simulink model "IEEE14_case"  (R2024b)
settings: Solver=FixedStepAuto  StartTime=0  StopTime=2  FixedStep=1e-7  RelTol=1e-3
values from neighbouring files (symbols this model uses):
  GFL_15_Bva = 0.009    [IEEE14_parameters.m]
  GFL_15_C_bus_pu = 7.179419    [IEEE14_parameters.m]
  GFL_15_f0 = 60    [IEEE14_parameters.m]
  GFL_15_I_id = 691.26967    [IEEE14_parameters.m]
  GFL_15_I_iq = 691.26967    [IEEE14_parameters.m]
  GFL_15_I_od = 45.2207    [IEEE14_parameters.m]
  GFL_15_I_oq = 45.2207    [IEEE14_parameters.m]
  GFL_15_I_pll = 0.78    [IEEE14_parameters.m]
  GFL_15_Kdi = 0.09    [IEEE14_parameters.m]
  GFL_15_Kdo = 0.9    [IEEE14_parameters.m]
  GFL_15_Kqi = 0.09    [IEEE14_parameters.m]
  GFL_15_Kqo = 0.9    [IEEE14_parameters.m]
  GFL_15_Lg_pu = 0.631447    [IEEE14_parameters.m]
  GFL_15_mode = 1    [IEEE14_parameters.m]
  GFL_15_P_id = 3.7166    [IEEE14_parameters.m]
  GFL_15_P_iq = 3.7166    [IEEE14_parameters.m]
  GFL_15_P_od = 0.4798    [IEEE14_parameters.m]
  GFL_15_P_oq = 0.4798    [IEEE14_parameters.m]
  GFL_15_P_pll = 290.42    [IEEE14_parameters.m]
  GFL_15_Qe_ref = 0.2    [IEEE14_parameters.m]
  GFL_15_Rg_pu = 0.024016    [IEEE14_parameters.m]
  GFL_15_Sbase = 1.000000e+4    (= 10000)    [IEEE14_parameters.m]
  GFL_15_Tdi = 0.01    [IEEE14_parameters.m]
  GFL_15_Tdo = 0.2    [IEEE14_parameters.m]
  GFL_15_Tqi = 0.01    [IEEE14_parameters.m]
  GFL_15_Tqo = 0.2    [IEEE14_parameters.m]
  GFL_15_Vbase = 380    [IEEE14_parameters.m]
  GFL_15_Vdc_ref = 1.011475    [IEEE14_parameters.m]
  GFL_15_Vdcbase = 700    [IEEE14_parameters.m]
  GFL_15_vq_ref = 0    [IEEE14_parameters.m]
  GFL_16_Bva = 0.002    [IEEE14_parameters.m]
  GFL_16_C_bus_pu = 7.179419    [IEEE14_parameters.m]
  GFL_16_f0 = 60    [IEEE14_parameters.m]
  GFL_16_I_id = 691.26967    [IEEE14_parameters.m]
  GFL_16_I_iq = 691.26967    [IEEE14_parameters.m]
  GFL_16_I_od = 45.2207    [IEEE14_parameters.m]
  GFL_16_I_oq = 45.2207    [IEEE14_parameters.m]
  GFL_16_I_pll = 0.78    [IEEE14_parameters.m]
  GFL_16_Kdi = 0.05    [IEEE14_parameters.m]
  GFL_16_Kdo = 0.5    [IEEE14_parameters.m]
  GFL_16_Kqi = 0.05    [IEEE14_parameters.m]
  GFL_16_Kqo = 0.5    [IEEE14_parameters.m]
  GFL_16_Lg_pu = 0.631447    [IEEE14_parameters.m]
  GFL_16_mode = 1    [IEEE14_parameters.m]
  GFL_16_P_id = 3.7166    [IEEE14_parameters.m]
  GFL_16_P_iq = 3.7166    [IEEE14_parameters.m]
  GFL_16_P_od = 0.4798    [IEEE14_parameters.m]
  GFL_16_P_oq = 0.4798    [IEEE14_parameters.m]
  GFL_16_P_pll = 290.42    [IEEE14_parameters.m]
  GFL_16_Qe_ref = 0.2    [IEEE14_parameters.m]
  GFL_16_Rg_pu = 0.024016    [IEEE14_parameters.m]
  GFL_16_Sbase = 1.000000e+4    (= 10000)    [IEEE14_parameters.m]
  GFL_16_Tdi = 0.01    [IEEE14_parameters.m]
  GFL_16_Tdo = 0.2    [IEEE14_parameters.m]
  GFL_16_Tqi = 0.01    [IEEE14_parameters.m]
  GFL_16_Tqo = 0.2    [IEEE14_parameters.m]
  GFL_16_Vbase = 380    [IEEE14_parameters.m]
  GFL_16_Vdc_ref = 1.01144    [IEEE14_parameters.m]
  GFL_16_Vdcbase = 700    [IEEE14_parameters.m]
  GFL_16_vq_ref = 0    [IEEE14_parameters.m]
  GFL_17_Bva = 0.002    [IEEE14_parameters.m]
  GFL_17_C_bus_pu = 7.179419    [IEEE14_parameters.m]
  GFL_17_f0 = 60    [IEEE14_parameters.m]
  GFL_17_I_id = 691.26967    [IEEE14_parameters.m]
  GFL_17_I_iq = 691.26967    [IEEE14_parameters.m]
  GFL_17_I_od = 45.2207    [IEEE14_parameters.m]
  GFL_17_I_oq = 45.2207    [IEEE14_parameters.m]
  GFL_17_I_pll = 0.78    [IEEE14_parameters.m]
  GFL_17_Kdi = 0.05    [IEEE14_parameters.m]
  GFL_17_Kdo = 0.5    [IEEE14_parameters.m]
  GFL_17_Kqi = 0.05    [IEEE14_parameters.m]
  GFL_17_Kqo = 0.5    [IEEE14_parameters.m]
  GFL_17_Lg_pu = 0.631447    [IEEE14_parameters.m]
  GFL_17_mode = 1    [IEEE14_parameters.m]
  GFL_17_P_id = 3.7166    [IEEE14_parameters.m]
  GFL_17_P_iq = 3.7166    [IEEE14_parameters.m]
  GFL_17_P_od = 0.4798    [IEEE14_parameters.m]
  GFL_17_P_oq = 0.4798    [IEEE14_parameters.m]
  GFL_17_P_pll = 290.42    [IEEE14_parameters.m]
  GFL_17_Qe_ref = 0.2    [IEEE14_parameters.m]
  GFL_17_Rg_pu = 0.024016    [IEEE14_parameters.m]
  GFL_17_Sbase = 1.000000e+4    (= 10000)    [IEEE14_parameters.m]
  GFL_17_Tdi = 0.01    [IEEE14_parameters.m]
  GFL_17_Tdo = 0.2    [IEEE14_parameters.m]
  GFL_17_Tqi = 0.01    [IEEE14_parameters.m]
  GFL_17_Tqo = 0.2    [IEEE14_parameters.m]
  GFL_17_Vbase = 380    [IEEE14_parameters.m]
  GFL_17_Vdc_ref = 1.011632    [IEEE14_parameters.m]
  GFL_17_Vdcbase = 700    [IEEE14_parameters.m]
  GFL_17_vq_ref = 0    [IEEE14_parameters.m]
  GFL_18_Bva = 0.002    [IEEE14_parameters.m]
  GFL_18_C_bus_pu = 7.179419    [IEEE14_parameters.m]
  GFL_18_f0 = 60    [IEEE14_parameters.m]
  GFL_18_I_id = 691.26967    [IEEE14_parameters.m]
  GFL_18_I_iq = 691.26967    [IEEE14_parameters.m]
  GFL_18_I_od = 45.2207    [IEEE14_parameters.m]
  GFL_18_I_oq = 45.2207    [IEEE14_parameters.m]
  GFL_18_I_pll = 0.78    [IEEE14_parameters.m]
  GFL_18_Kdi = 0.05    [IEEE14_parameters.m]
  GFL_18_Kdo = 0.5    [IEEE14_parameters.m]
  GFL_18_Kqi = 0.05    [IEEE14_parameters.m]
  GFL_18_Kqo = 0.5    [IEEE14_parameters.m]
  GFL_18_Lg_pu = 0.631447    [IEEE14_parameters.m]
  GFL_18_mode = 1    [IEEE14_parameters.m]
  GFL_18_P_id = 3.7166    [IEEE14_parameters.m]
  GFL_18_P_iq = 3.7166    [IEEE14_parameters.m]
  GFL_18_P_od = 0.4798    [IEEE14_parameters.m]
  GFL_18_P_oq = 0.4798    [IEEE14_parameters.m]
  GFL_18_P_pll = 290.42    [IEEE14_parameters.m]
  GFL_18_Qe_ref = 0.2    [IEEE14_parameters.m]
  GFL_18_Rg_pu = 0.024016    [IEEE14_parameters.m]
  GFL_18_Sbase = 1.000000e+4    (= 10000)    [IEEE14_parameters.m]
  GFL_18_Tdi = 0.01    [IEEE14_parameters.m]
  GFL_18_Tdo = 0.2    [IEEE14_parameters.m]
  GFL_18_Tqi = 0.01    [IEEE14_parameters.m]
  GFL_18_Tqo = 0.2    [IEEE14_parameters.m]
  GFL_18_Vbase = 380    [IEEE14_parameters.m]
  GFL_18_Vdc_ref = 1.011572    [IEEE14_parameters.m]
  GFL_18_Vdcbase = 700    [IEEE14_parameters.m]
  GFL_18_vq_ref = 0    [IEEE14_parameters.m]
  ... (+180 more)
(part 13 of 25)

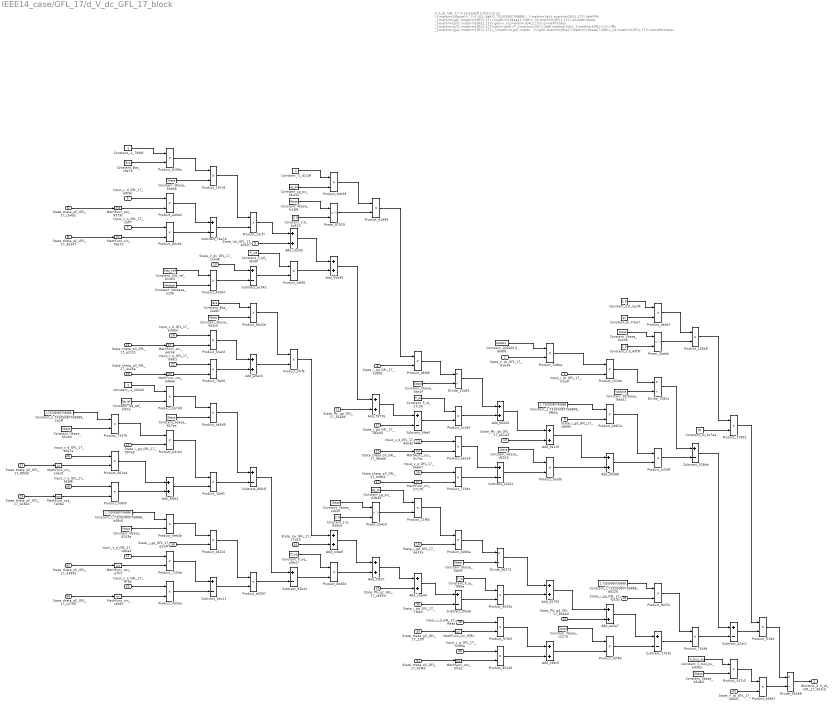
== system IEEE14_case/GFL_17/d_V_dc_GFL_17_block ==
  note: d_V_dc_GFL_17 in case14gfl
      | $-\frac{2\,\pi \,{\mathrm{Vbase}}^2\,f_{0}\,\left(1.73205080756888\,i_{\mathrm{gd},\mathrm{GFL},17}\,\left(\Phi _{\mathrm{gb},\mathrm{GFL},17}+\mathrm{Vbase}\,\left(v_{d,\mathrm{GFL},17}\,\cos\left(\theta _{\mathrm{pll},\mathrm{GFL},17}\right)-v_{q,\mathrm{GFL},17}\,\sin\left(\theta _{\mathrm{pll},\mathrm{GFL},17}\right)\right)+P_{\mathrm{id}}\,\left(\mathrm{Idv}_{\mathrm{GFL},17}+\Phi _{\mathrm{ga},\mathrm{GFL},17}-i_{\mathrm{gd},\mathrm{GFL},17}+P_{\mathrm{od}}\,\left(V_{\mathrm{dc},\mathrm{GFL},17}-\mathrm{Vdcbase}\,\mathrm{Vdc}_{\mathrm{ref}}\right)-\mathrm{Bva}\,\mathrm{Vbase}\,\left(v_{d,\mathrm{GFL},17}\,\cos\left(\theta _{\mathrm{pll},\mathrm{GFL},17}\right)-v_{q,\mathrm{GFL},17}\,\sin\left(\theta _{\mathrm{pll},\mathrm{GFL},17}\right)\right)\right)-\frac{\mathrm{Lg}_{\mathrm{pu}}\,{\mathrm{Vbase}}^2\,i_{\mathrm{gq},\mathrm{GFL},17}}{\mathrm{Sbase}}\right)+1.73205080756888\,i_{\mathrm{gq},\mathrm{GFL},17}\,\left(\Phi _{\mathrm{gd},\mathrm{GFL},17}-\mathrm{Vbase}\,\left(v_{q,\mathrm{GFL},17}\,\cos\left(\theta _{\mathrm{pll},\mathrm{GFL},17}\right)+v_{d,\mathrm{GFL},17}\,\sin\left(\theta _{\mathrm{pll},\mathrm{GFL},17}\right)\right)+P_{\mathrm{iq}}\,\left(\mathrm{Iqv}_{\mathrm{GFL},17}+\Phi _{\mathrm{gc},\mathrm{GFL},17}-i_{\mathrm{gq},\mathrm{GFL},17}-P_{\mathrm{oq}}\,\left(\mathrm{Qe}_{\mathrm{ref}}\,\mathrm{Sbase}+1.73205080756888\,\mathrm{Vbase}\,i_{\mathrm{gd},\mathrm{GFL},17}\,\left(v_{q,\mathrm{GFL},17}\,\cos\left(\theta _{\mathrm{pll},\mathrm{GFL},17}\right)+v_{d,\mathrm{GFL},17}\,\sin\left(\theta _{\mathrm{pll},\mathrm{GFL},17}\right)\right)+1.73205080756888\,\mathrm{Vbase}\,i_{\mathrm{gq},\mathrm{GFL},17}\,\left(v_{d,\mathrm{GFL},17}\,\cos\left(\theta _{\mathrm{pll},\mathrm{GFL},17}\right)-v_{q,\mathrm{GFL},17}\,\sin\left(\theta _{\mathrm{pll},\mathrm{GFL},17}\right)\right)\right)+\mathrm{Bva}\,\mathrm{Vbase}\,\left(v_{q,\mathrm{GFL},17}\,\cos\left(\theta _{\mathrm{pll},\mathrm{GFL},17}\right)+v_{d,\mathrm{GFL},17}\,\sin\left(\theta _{\mathrm{pll},\mathrm{GFL},17}\right)\right)\right)+\frac{\mathrm{Lg}_{\mathrm{pu}}\,{\mathrm{Vbase}}^2\,i_{\mathrm{gd},\mathrm{GFL},17}}{\mathrm{Sbase}}\right)-\frac{100000.0\,V_{\mathrm{dc},\mathrm{GFL},17}\,i_{\mathrm{dc},\mathrm{GFL},17}}{\mathrm{Vdcbase}}\right)}{C_{\mathrm{bus},\mathrm{pu}}\,\mathrm{Sbase}\,V_{\mathrm{dc},\mathrm{GFL},17}}$
      | Automatically generated on 2025-10-09 21:36:53 .
  State_V_dc_GFL_17_61ba6 : Inport
  Input_i_dc_GFL_17_b2e3f : Inport  Port=2
  State_i_gd_GFL_17_c8e95 : Inport  Port=3
  State_i_gq_GFL_17_13802 : Inport  Port=4
  Input_v_d_GFL_17_69f5b : Inport  Port=5
  State_theta_pll_GFL_17_ce4a2 : Inport  Port=6
  Input_v_q_GFL_17_2aff7 : Inport  Port=7
  State_theta_pll_GFL_17_4a347 : Inport  Port=8
  State_Idv_GFL_17_e3537 : Inport  Port=9
  State_V_dc_GFL_17_1c4d8 : Inport  Port=10
  State_Phi_ga_GFL_17_55e9b : Inport  Port=11
  State_i_gd_GFL_17_9e4d0 : Inport  Port=12
  State_Phi_gb_GFL_17_a014d : Inport  Port=13
  Input_v_d_GFL_17_85bd5 : Inport  Port=14
  State_theta_pll_GFL_17_9bdeb : Inport  Port=15
  Input_v_q_GFL_17_0e6b7 : Inport  Port=16
  State_theta_pll_GFL_17_bd8c4 : Inport  Port=17
  State_i_gq_GFL_17_f2530 : Inport  Port=18
  State_i_gd_GFL_17_ee33a : Inport  Port=19
  Input_v_d_GFL_17_e38bd : Inport  Port=20
  State_theta_pll_GFL_17_e2101 : Inport  Port=21
  Input_v_q_GFL_17_b68cc : Inport  Port=22
  State_theta_pll_GFL_17_4c26e : Inport  Port=23
  State_Iqv_GFL_17_27d19 : Inport  Port=24
  State_i_gd_GFL_17_097e8 : Inport  Port=25
  Input_v_d_GFL_17_4b47a : Inport  Port=26
  State_theta_pll_GFL_17_8f50d : Inport  Port=27
  Input_v_q_GFL_17_959f8 : Inport  Port=28
  State_theta_pll_GFL_17_b2824 : Inport  Port=29
  State_i_gq_GFL_17_e224f : Inport  Port=30
  Input_v_d_GFL_17_cb6ad : Inport  Port=31
  State_theta_pll_GFL_17_43992 : Inport  Port=32
  Input_v_q_GFL_17_ff76b : Inport  Port=33
  State_theta_pll_GFL_17_c2799 : Inport  Port=34
  State_Phi_gc_GFL_17_ca63d : Inport  Port=35
  State_i_gq_GFL_17_7fe40 : Inport  Port=36
  State_Phi_gd_GFL_17_8444d : Inport  Port=37
  Input_v_d_GFL_17_ffaea : Inport  Port=38
  State_theta_pll_GFL_17_12fff : Inport  Port=39
  Input_v_q_GFL_17_0295a : Inport  Port=40
  State_theta_pll_GFL_17_03f60 : Inport  Port=41
  State_V_dc_GFL_17_4d001 : Inport  Port=42
  Add_0602b : Sum
  Add_1ae44 : Sum
  Add_1b26b : Sum
  Add_2fb64 : Sum
  Add_3f927 : Sum
  Add_45706 : Sum
  Add_55a95 : Sum
  Add_79776 : Sum
  Add_9410f : Sum
  Add_a9ec0 : Sum
  Add_aa5a7 : Sum
  Add_c38c5 : Sum
  Add_cc8e9 : Sum
  Add_d0388 : Sum
  Constant_-1_202e6 : Constant  Value=-1
  Constant_-1_79dbf : Constant  Value=-1
  Constant_-1_d11df : Constant  Value=-1
  Constant_1.73205080756888_2a2ff : Constant  Value=1.73205080756888
  Constant_1.73205080756888_8fb5a : Constant  Value=1.73205080756888
  Constant_1.73205080756888_b48c8 : Constant  Value=1.73205080756888
  Constant_1.73205080756888_d6226 : Constant  Value=1.73205080756888
  Constant_100000.0_8b8f6 : Constant  Value=100000.0
  Constant_2.0_1ecf4 : Constant  Value=2.0
  Constant_2.0_4a610 : Constant  Value=2.0
  Constant_2.0_4df9f : Constant  Value=2.0
  Constant_2.0_940b0 : Constant  Value=2.0
  Constant_Bva_2ee87 : Constant  Value=Bva
  Constant_Bva_c9e76 : Constant  Value=Bva
  Constant_C_bus_pu_e43b5 : Constant  Value=C_bus_pu
  Constant_Lg_pu_63ba9 : Constant  Value=Lg_pu
  Constant_Lg_pu_6b432 : Constant  Value=Lg_pu
  Constant_P_id_27c3b : Constant  Value=P_id
  Constant_P_iq_7f96e : Constant  Value=P_iq
  Constant_P_od_4b38f : Constant  Value=P_od
  Constant_P_oq_a9b47 : Constant  Value=P_oq
  Constant_Qe_ref_ef57e : Constant  Value=Qe_ref
  Constant_Sbase_6bbf3 : Constant  Value=Sbase
  Constant_Sbase_847ea : Constant  Value=Sbase
  Constant_Sbase_b5ded : Constant  Value=Sbase
  Constant_Sbase_bba4f : Constant  Value=Sbase
  Constant_Vbase_0c438 : Constant  Value=Vbase
  Constant_Vbase_5bab8 : Constant  Value=Vbase
  Constant_Vbase_6243e : Constant  Value=Vbase
  Constant_Vbase_904c0 : Constant  Value=Vbase
  Constant_Vbase_b14f6 : Constant  Value=Vbase
  Constant_Vbase_b5c4d : Constant  Value=Vbase
  Constant_Vbase_c2279 : Constant  Value=Vbase
  Constant_Vbase_ccb00 : Constant  Value=Vbase
  Constant_Vbase_d0024 : Constant  Value=Vbase
  Constant_Vdc_ref_b1363 : Constant  Value=Vdc_ref
  Constant_Vdcbase_9dd31 : Constant  Value=Vdcbase
  Constant_Vdcbase_cc5f6 : Constant  Value=Vdcbase
  Constant_f0_3a7aa : Constant  Value=f0
  Constant_pi_7dce7 : Constant  Value=pi
  Divide_03d52 : Product  Inputs=*/
  Divide_46488 : Product  Inputs=*/
  Divide_7582a : Product  Inputs=*/
  Divide_96273 : Product  Inputs=*/
  MathFunc_cos_0fca1 : Trigonometry  Operator=cos
  MathFunc_cos_546b6 : Trigonometry  Operator=cos
  MathFunc_cos_5c7dc : Trigonometry  Operator=cos
  MathFunc_cos_7e0be : Trigonometry  Operator=cos
  MathFunc_cos_8379c : Trigonometry  Operator=cos
  MathFunc_cos_e7fcf : Trigonometry  Operator=cos
  MathFunc_sin_1dec9 : Trigonometry
  MathFunc_sin_27178 : Trigonometry
  MathFunc_sin_76e72 : Trigonometry
  MathFunc_sin_a4cb6 : Trigonometry
  MathFunc_sin_c4b6f : Trigonometry
  MathFunc_sin_f3f5c : Trigonometry
  Power_2b4a3 : Math  Operator=pow
  Power_3bebb : Math  Operator=pow
  Power_87029 : Math  Operator=pow
  Product_006f3 : Product
  Product_00d6d : Product
  Product_0d3aa : Product
  Product_158a8 : Product
  Product_17903 : Product
  Product_197c9 : Product
  Product_21f94 : Product
  Product_23cf7 : Product
  Product_2fcf6 : Product
  Product_33ef1 : Product
  Product_347c5 : Product
  Product_400b7 : Product
  Product_401ed : Product
  Product_557d9 : Product
  Product_6196a : Product
  Product_6b42e : Product
  Product_6c3bf : Product
  Product_7153e : Product
  Product_719bc : Product
  Product_7337b : Product
  Product_74c9d : Product
  Product_7b8be : Product
  Product_7feb9 : Product
  Product_85149 : Product
  Product_89c94 : Product
  Product_9625b : Product
  Product_9705f : Product
  Product_b080a : Product
  Product_b318f : Product
  Product_b3c64 : Product
  Product_b484f : Product
  Product_bb814 : Product
  Product_bcb09 : Product
  Product_be2e5 : Product
  Product_c21bb : Product
  Product_c4f46 : Product
  Product_c8216 : Product
  Product_d6fd9 : Product
  Product_da9d9 : Product
  Product_de8a7 : Product
  Product_e1d99 : Product
  Product_e49a5 : Product
  Product_e9267 : Product
  Product_eee2b : Product
  Product_f2e2d : Product
  Product_f7c94 : Product
  Product_fa3db : Product
  Product_fb253 : Product
  Product_fd780 : Product
  Subtract_14521 : Sum  Inputs=+-
  Subtract_1753b : Sum  Inputs=+-
  Subtract_328da : Sum  Inputs=+-
  Subtract_42ac1 : Sum  Inputs=+-
  Subtract_4ac11 : Sum  Inputs=+-
  Subtract_74e74 : Sum  Inputs=+-
  Subtract_95b41 : Sum  Inputs=+-
  Subtract_9fde7 : Sum  Inputs=+-
  Subtract_d0b2f : Sum  Inputs=+-
  Subtract_ecb42 : Sum  Inputs=+-
  Subtract_f05a8 : Sum  Inputs=+-
  Blockout_d_V_dc_GFL_17_353cb : Outport
  wires:
  Product_7b8be/1 -> Product_c21bb/1
  Input_v_q_GFL_17_ff76b/1 -> Product_0d3aa/1
  Subtract_f05a8/1 -> Product_9625b/2
  Divide_46488/1 -> Blockout_d_V_dc_GFL_17_353cb/1
  Constant_Sbase_b5ded/1 -> Product_347c5/2
  Add_9410f/1 -> Add_d0388/1
  State_theta_pll_GFL_17_4c26e/1 -> MathFunc_cos_546b6/1
  Product_347c5/1 -> Product_b484f/1
  Constant_C_bus_pu_e43b5/1 -> Product_347c5/1
  State_i_gq_GFL_17_f2530/1 -> Product_fb253/2
  Product_0d3aa/1 -> Subtract_4ac11/2
  Input_v_q_GFL_17_b68cc/1 -> Product_7feb9/1
  Add_d0388/1 -> Product_b318f/2
  Product_b484f/1 -> Divide_46488/2
  Constant_1.73205080756888_b48c8/1 -> Product_eee2b/1
  Product_eee2b/1 -> Product_c8216/1
  Product_74c9d/1 -> Subtract_42ac1/2
  State_Phi_gc_GFL_17_ca63d/1 -> Add_1ae44/2
  State_theta_pll_GFL_17_b2824/1 -> MathFunc_cos_7e0be/1
  Input_v_q_GFL_17_0e6b7/1 -> Product_719bc/1
  Constant_Vdcbase_cc5f6/1 -> Product_400b7/2
  MathFunc_cos_7e0be/1 -> Product_006f3/2
  Constant_Vbase_b5c4d/1 -> Product_7337b/2
  State_theta_pll_GFL_17_bd8c4/1 -> MathFunc_sin_27178/1
  Product_6196a/1 -> Product_197c9/1
  State_V_dc_GFL_17_4d001/1 -> Product_b484f/2
  Product_f7c94/1 -> Divide_46488/1
  State_theta_pll_GFL_17_43992/1 -> MathFunc_cos_e7fcf/1
  State_V_dc_GFL_17_1c4d8/1 -> Subtract_ecb42/1
  Divide_96273/1 -> Add_45706/1
  MathFunc_cos_e7fcf/1 -> Product_7153e/2
  MathFunc_sin_c4b6f/1 -> Product_0d3aa/2
  Constant_Vbase_6243e/1 -> Product_eee2b/2
  Subtract_42ac1/1 -> Product_f7c94/2
  State_theta_pll_GFL_17_c2799/1 -> MathFunc_sin_c4b6f/1
  Power_87029/1 -> Product_e1d99/2
  Subtract_d0b2f/1 -> Subtract_95b41/1
  Subtract_4ac11/1 -> Product_e9267/2
  Subtract_1753b/1 -> Product_74c9d/2
  Product_33ef1/1 -> Subtract_d0b2f/2
  Add_1ae44/1 -> Subtract_f05a8/1
  Constant_Vbase_c2279/1 -> Product_fd780/1
  Product_fd780/1 -> Subtract_1753b/2
  Add_c38c5/1 -> Product_fd780/2
  Input_v_q_GFL_17_0295a/1 -> Product_85149/1
  Product_85149/1 -> Add_c38c5/2
  State_theta_pll_GFL_17_03f60/1 -> MathFunc_cos_0fca1/1
  MathFunc_cos_0fca1/1 -> Product_85149/2
  State_theta_pll_GFL_17_8f50d/1 -> MathFunc_sin_1dec9/1
  State_i_gd_GFL_17_9e4d0/1 -> Subtract_9fde7/2
  Product_e9267/1 -> Subtract_95b41/2
  Constant_Vbase_d0024/1 -> Product_fa3db/1
  Add_2fb64/1 -> Product_33ef1/2
  Product_c21bb/1 -> Divide_7582a/1
  State_theta_pll_GFL_17_12fff/1 -> MathFunc_sin_f3f5c/1
  Input_v_d_GFL_17_ffaea/1 -> Product_9705f/1
  Product_9705f/1 -> Add_c38c5/1
  Product_de8a7/1 -> Product_158a8/1
  Product_c8216/1 -> Product_e9267/1
  MathFunc_sin_f3f5c/1 -> Product_9705f/2
  State_i_gq_GFL_17_e224f/1 -> Product_c8216/2
  Constant_2.0_940b0/1 -> Power_2b4a3/2
  Product_c4f46/1 -> Add_55a95/2
  Subtract_14521/1 -> Product_fa3db/2
  MathFunc_sin_1dec9/1 -> Product_401ed/2
  Input_v_d_GFL_17_cb6ad/1 -> Product_7153e/1
  Product_7153e/1 -> Subtract_4ac11/1
  Add_aa5a7/1 -> Subtract_1753b/1
  State_Phi_gd_GFL_17_8444d/1 -> Add_aa5a7/2
  Add_45706/1 -> Add_aa5a7/1
  Product_9625b/1 -> Add_45706/2
  Constant_Lg_pu_6b432/1 -> Product_bcb09/2
  State_i_gq_GFL_17_7fe40/1 -> Subtract_f05a8/2
  Add_3f927/1 -> Add_1ae44/1
  Product_00d6d/1 -> Add_3f927/2
  Subtract_95b41/1 -> Product_00d6d/2
  Product_7337b/1 -> Product_b3c64/1
  State_Idv_GFL_17_e3537/1 -> Add_1b26b/2
  Input_v_q_GFL_17_959f8/1 -> Product_006f3/1
  Product_006f3/1 -> Add_2fb64/2
  Product_719bc/1 -> Subtract_14521/2
  Input_v_d_GFL_17_4b47a/1 -> Product_401ed/1
  Product_401ed/1 -> Add_2fb64/1
  Product_b318f/1 -> Subtract_328da/2
  Product_b3c64/1 -> Product_33ef1/1
  State_Phi_gb_GFL_17_a014d/1 -> Add_9410f/2
  State_i_gd_GFL_17_097e8/1 -> Product_b3c64/2
  Constant_2.0_4df9f/1 -> Power_3bebb/2
  Constant_1.73205080756888_2a2ff/1 -> Product_7337b/1
  Constant_Qe_ref_ef57e/1 -> Product_557d9/2
  Product_da9d9/1 -> Subtract_d0b2f/1
  Subtract_ecb42/1 -> Product_c4f46/2
  Constant_Sbase_847ea/1 -> Product_da9d9/2
  Product_557d9/1 -> Product_da9d9/1
  Constant_Vdcbase_9dd31/1 -> Divide_7582a/2
  Constant_-1_202e6/1 -> Product_557d9/1
  Constant_P_oq_a9b47/1 -> Product_00d6d/1
  Add_cc8e9/1 -> Add_3f927/1
  State_Iqv_GFL_17_27d19/1 -> Add_cc8e9/2
  Product_2fcf6/1 -> Add_cc8e9/1
  Add_a9ec0/1 -> Product_2fcf6/2
  Product_7feb9/1 -> Add_a9ec0/2
  MathFunc_cos_546b6/1 -> Product_7feb9/2
  Product_f2e2d/1 -> Add_a9ec0/1
  MathFunc_sin_a4cb6/1 -> Product_f2e2d/2
  State_theta_pll_GFL_17_e2101/1 -> MathFunc_sin_a4cb6/1
  Input_v_d_GFL_17_e38bd/1 -> Product_f2e2d/1
  Product_6b42e/1 -> Product_2fcf6/1
  Constant_Vbase_904c0/1 -> Product_6b42e/2
  Constant_Bva_2ee87/1 -> Product_6b42e/1
  Constant_P_iq_7f96e/1 -> Product_9625b/1
  Input_i_dc_GFL_17_b2e3f/1 -> Product_c21bb/2
  Constant_Sbase_6bbf3/1 -> Divide_96273/2
  Product_b080a/1 -> Divide_96273/1
  State_i_gd_GFL_17_ee33a/1 -> Product_b080a/2
  Constant_Vdc_ref_b1363/1 -> Product_400b7/1
  Product_21f94/1 -> Product_b080a/1
  State_i_gd_GFL_17_c8e95/1 -> Product_bb814/2
  Power_2b4a3/1 -> Product_21f94/2
  State_theta_pll_GFL_17_4a347/1 -> MathFunc_sin_76e72/1
  Product_fb253/1 -> Product_74c9d/1
  Constant_Vbase_ccb00/1 -> Power_2b4a3/1
  Constant_Lg_pu_63ba9/1 -> Product_21f94/1
  Constant_1.73205080756888_d6226/1 -> Product_fb253/1
  Subtract_328da/1 -> Subtract_42ac1/1
  Constant_f0_3a7aa/1 -> Product_17903/2
  Product_fa3db/1 -> Add_d0388/2
  MathFunc_sin_27178/1 -> Product_719bc/2
  MathFunc_cos_5c7dc/1 -> Product_be2e5/2
  Product_be2e5/1 -> Subtract_14521/1
  Subtract_74e74/1 -> Product_23cf7/2
  State_theta_pll_GFL_17_9bdeb/1 -> MathFunc_cos_5c7dc/1
  Input_v_d_GFL_17_85bd5/1 -> Product_be2e5/1
  Add_0602b/1 -> Add_9410f/1
  Product_6c3bf/1 -> Add_0602b/2
  Subtract_9fde7/1 -> Product_6c3bf/2
  Add_79776/1 -> Subtract_9fde7/1
  State_Phi_ga_GFL_17_55e9b/1 -> Add_79776/2
  Add_55a95/1 -> Add_79776/1
  Product_400b7/1 -> Subtract_ecb42/2
  Constant_P_od_4b38f/1 -> Product_c4f46/1
  Add_1b26b/1 -> Add_55a95/1
  Product_23cf7/1 -> Add_1b26b/1
  Product_89c94/1 -> Subtract_74e74/2
  MathFunc_sin_76e72/1 -> Product_89c94/2
  Input_v_q_GFL_17_2aff7/1 -> Product_89c94/1
  Product_e49a5/1 -> Subtract_74e74/1
  MathFunc_cos_8379c/1 -> Product_e49a5/2
  State_theta_pll_GFL_17_ce4a2/1 -> MathFunc_cos_8379c/1
  Input_v_d_GFL_17_69f5b/1 -> Product_e49a5/1
  Constant_Vbase_0c438/1 -> Power_3bebb/1
  Product_197c9/1 -> Product_23cf7/1
  Constant_Vbase_5bab8/1 -> Product_197c9/2
  Constant_Bva_c9e76/1 -> Product_6196a/2
  Constant_-1_79dbf/1 -> Product_6196a/1
  Constant_P_id_27c3b/1 -> Product_6c3bf/1
  Divide_03d52/1 -> Add_0602b/1
  Constant_Sbase_bba4f/1 -> Divide_03d52/2
  Product_d6fd9/1 -> Divide_03d52/1
  State_i_gq_GFL_17_13802/1 -> Product_d6fd9/2
  Product_e1d99/1 -> Product_d6fd9/1
  Constant_2.0_4a610/1 -> Power_87029/2
  Constant_Vbase_b14f6/1 -> Power_87029/1
  Product_bcb09/1 -> Product_e1d99/1
  Constant_-1_d11df/1 -> Product_bcb09/1
  Product_bb814/1 -> Product_b318f/1
  Constant_1.73205080756888_8fb5a/1 -> Product_bb814/1
  Divide_7582a/1 -> Subtract_328da/1
  State_V_dc_GFL_17_61ba6/1 -> Product_7b8be/2
  Constant_100000.0_8b8f6/1 -> Product_7b8be/1
  Product_17903/1 -> Product_f7c94/1
  Product_158a8/1 -> Product_17903/1
  Power_3bebb/1 -> Product_158a8/2
  Constant_pi_7dce7/1 -> Product_de8a7/2
  Constant_2.0_1ecf4/1 -> Product_de8a7/1

== system IEEE14_case/GFL_17/d_i_gd_GFL_17_block ==
  note: d_i_gd_GFL_17 in case14gfl
      | $\frac{2\,\pi \,\mathrm{Sbase}\,f_{0}\,\left(\Phi _{\mathrm{gb},\mathrm{GFL},17}+P_{\mathrm{id}}\,\left(\mathrm{Idv}_{\mathrm{GFL},17}+\Phi _{\mathrm{ga},\mathrm{GFL},17}-i_{\mathrm{gd},\mathrm{GFL},17}+P_{\mathrm{od}}\,\left(V_{\mathrm{dc},\mathrm{GFL},17}-\mathrm{Vdcbase}\,\mathrm{Vdc}_{\mathrm{ref}}\right)-\mathrm{Bva}\,\mathrm{Vbase}\,\left(v_{d,\mathrm{GFL},17}\,\cos\left(\theta _{\mathrm{pll},\mathrm{GFL},17}\right)-v_{q,\mathrm{GFL},17}\,\sin\left(\theta _{\mathrm{pll},\mathrm{GFL},17}\right)\right)\right)-\frac{\mathrm{Rg}_{\mathrm{pu}}\,{\mathrm{Vbase}}^2\,i_{\mathrm{gd},\mathrm{GFL},17}}{\mathrm{Sbase}}\right)}{\mathrm{Lg}_{\mathrm{pu}}\,{\mathrm{Vbase}}^2}$
      | Automatically generated on 2025-10-09 21:36:35 .
  Input_v_d_GFL_17_f609b : Inport
  State_theta_pll_GFL_17_c766c : Inport  Port=2
  Input_v_q_GFL_17_15e66 : Inport  Port=3
  State_theta_pll_GFL_17_748be : Inport  Port=4
  State_Idv_GFL_17_31090 : Inport  Port=5
  State_V_dc_GFL_17_0edd3 : Inport  Port=6
  State_Phi_ga_GFL_17_11b44 : Inport  Port=7
  State_i_gd_GFL_17_ac7fa : Inport  Port=8
  State_Phi_gb_GFL_17_45475 : Inport  Port=9
  State_i_gd_GFL_17_d59fc : Inport  Port=10
  Add_4dbcd : Sum
  Add_ade08 : Sum
  Add_d6e4f : Sum
  Add_e1609 : Sum
  Constant_-1_c5e7d : Constant  Value=-1
  Constant_2.0_0f4b2 : Constant  Value=2.0
  Constant_2.0_54c24 : Constant  Value=2.0
  Constant_2.0_c0832 : Constant  Value=2.0
  Constant_Bva_cd769 : Constant  Value=Bva
  Constant_Lg_pu_c7d28 : Constant  Value=Lg_pu
  Constant_P_id_541e3 : Constant  Value=P_id
  Constant_P_od_79a8b : Constant  Value=P_od
  Constant_Rg_pu_e6839 : Constant  Value=Rg_pu
  Constant_Sbase_eb741 : Constant  Value=Sbase
  Constant_Sbase_f5482 : Constant  Value=Sbase
  Constant_Vbase_2eb24 : Constant  Value=Vbase
  Constant_Vbase_692de : Constant  Value=Vbase
  Constant_Vbase_f0ed1 : Constant  Value=Vbase
  Constant_Vdc_ref_63d9b : Constant  Value=Vdc_ref
  Constant_Vdcbase_df9b1 : Constant  Value=Vdcbase
  Constant_f0_ee6e5 : Constant  Value=f0
  Constant_pi_5d07d : Constant  Value=pi
  Divide_0eb56 : Product  Inputs=*/
  Divide_55667 : Product  Inputs=*/
  MathFunc_cos_b4f71 : Trigonometry  Operator=cos
  MathFunc_sin_1fc48 : Trigonometry
  Power_502a3 : Math  Operator=pow
  Power_ce599 : Math  Operator=pow
  Product_08af4 : Product
  Product_3efe8 : Product
  Product_63297 : Product
  Product_79c66 : Product
  Product_7ee29 : Product
  Product_86d34 : Product
  Product_980f7 : Product
  Product_a32e4 : Product
  Product_c9580 : Product
  Product_c9b9a : Product
  Product_e4418 : Product
  Product_e8224 : Product
  Product_f2f6a : Product
  Product_fb0f8 : Product
  Product_fdaaa : Product
  Subtract_15659 : Sum  Inputs=+-
  Subtract_93eda : Sum  Inputs=+-
  Subtract_a421d : Sum  Inputs=+-
  Subtract_cf3c5 : Sum  Inputs=+-
  Blockout_d_i_gd_GFL_17_06168 : Outport
  wires:
  State_theta_pll_GFL_17_c766c/1 -> MathFunc_cos_b4f71/1
  MathFunc_cos_b4f71/1 -> Product_86d34/2
  Subtract_a421d/1 -> Product_c9580/2
  Constant_Bva_cd769/1 -> Product_7ee29/2
  State_theta_pll_GFL_17_748be/1 -> MathFunc_sin_1fc48/1
  Constant_Vbase_2eb24/1 -> Product_c9b9a/2
  Constant_-1_c5e7d/1 -> Product_7ee29/1
  Input_v_d_GFL_17_f609b/1 -> Product_86d34/1
  Input_v_q_GFL_17_15e66/1 -> Product_fdaaa/1
  State_Phi_gb_GFL_17_45475/1 -> Add_d6e4f/2
  MathFunc_sin_1fc48/1 -> Product_fdaaa/2
  Product_7ee29/1 -> Product_c9b9a/1
  Product_86d34/1 -> Subtract_a421d/1
  Product_fdaaa/1 -> Subtract_a421d/2
  Divide_55667/1 -> Blockout_d_i_gd_GFL_17_06168/1
  Constant_Vdc_ref_63d9b/1 -> Product_e4418/1
  State_V_dc_GFL_17_0edd3/1 -> Subtract_93eda/1
  Constant_Vdcbase_df9b1/1 -> Product_e4418/2
  Product_c9b9a/1 -> Product_c9580/1
  Product_e4418/1 -> Subtract_93eda/2
  Product_c9580/1 -> Add_e1609/1
  State_Idv_GFL_17_31090/1 -> Add_e1609/2
  State_Phi_ga_GFL_17_11b44/1 -> Add_4dbcd/2
  Constant_P_od_79a8b/1 -> Product_e8224/1
  Subtract_93eda/1 -> Product_e8224/2
  Add_e1609/1 -> Add_ade08/1
  Product_e8224/1 -> Add_ade08/2
  Add_ade08/1 -> Add_4dbcd/1
  Constant_2.0_54c24/1 -> Power_ce599/2
  Constant_Vbase_f0ed1/1 -> Power_ce599/1
  Add_4dbcd/1 -> Subtract_cf3c5/1
  State_i_gd_GFL_17_ac7fa/1 -> Subtract_cf3c5/2
  Product_79c66/1 -> Product_fb0f8/1
  Constant_Rg_pu_e6839/1 -> Product_79c66/1
  Power_ce599/1 -> Product_79c66/2
  Constant_Sbase_eb741/1 -> Product_3efe8/2
  Product_a32e4/1 -> Product_3efe8/1
  Constant_2.0_0f4b2/1 -> Product_a32e4/1
  Product_3efe8/1 -> Product_63297/1
  Constant_pi_5d07d/1 -> Product_a32e4/2
  Product_f2f6a/1 -> Add_d6e4f/1
  Constant_P_id_541e3/1 -> Product_f2f6a/1
  Subtract_cf3c5/1 -> Product_f2f6a/2
  State_i_gd_GFL_17_d59fc/1 -> Product_fb0f8/2
  Product_fb0f8/1 -> Divide_0eb56/1
  Product_08af4/1 -> Divide_55667/2
  Constant_Sbase_f5482/1 -> Divide_0eb56/2
  Constant_f0_ee6e5/1 -> Product_63297/2
  Add_d6e4f/1 -> Subtract_15659/1
  Divide_0eb56/1 -> Subtract_15659/2
  Power_502a3/1 -> Product_08af4/2
  Constant_Vbase_692de/1 -> Power_502a3/1
  Constant_2.0_c0832/1 -> Power_502a3/2
  Product_63297/1 -> Product_980f7/1
  Subtract_15659/1 -> Product_980f7/2
  Constant_Lg_pu_c7d28/1 -> Product_08af4/1
  Product_980f7/1 -> Divide_55667/1

== system IEEE14_case/GFL_17/d_i_gq_GFL_17_block ==
  note: d_i_gq_GFL_17 in case14gfl
      | $\frac{2\,\pi \,\mathrm{Sbase}\,f_{0}\,\left(\Phi _{\mathrm{gd},\mathrm{GFL},17}+P_{\mathrm{iq}}\,\left(\mathrm{Iqv}_{\mathrm{GFL},17}+\Phi _{\mathrm{gc},\mathrm{GFL},17}-i_{\mathrm{gq},\mathrm{GFL},17}-P_{\mathrm{oq}}\,\left(\mathrm{Qe}_{\mathrm{ref}}\,\mathrm{Sbase}+1.73205080756888\,\mathrm{Vbase}\,i_{\mathrm{gd},\mathrm{GFL},17}\,\left(v_{q,\mathrm{GFL},17}\,\cos\left(\theta _{\mathrm{pll},\mathrm{GFL},17}\right)+v_{d,\mathrm{GFL},17}\,\sin\left(\theta _{\mathrm{pll},\mathrm{GFL},17}\right)\right)+1.73205080756888\,\mathrm{Vbase}\,i_{\mathrm{gq},\mathrm{GFL},17}\,\left(v_{d,\mathrm{GFL},17}\,\cos\left(\theta _{\mathrm{pll},\mathrm{GFL},17}\right)-v_{q,\mathrm{GFL},17}\,\sin\left(\theta _{\mathrm{pll},\mathrm{GFL},17}\right)\right)\right)+\mathrm{Bva}\,\mathrm{Vbase}\,\left(v_{q,\mathrm{GFL},17}\,\cos\left(\theta _{\mathrm{pll},\mathrm{GFL},17}\right)+v_{d,\mathrm{GFL},17}\,\sin\left(\theta _{\mathrm{pll},\mathrm{GFL},17}\right)\right)\right)-\frac{\mathrm{Rg}_{\mathrm{pu}}\,{\mathrm{Vbase}}^2\,i_{\mathrm{gq},\mathrm{GFL},17}}{\mathrm{Sbase}}\right)}{\mathrm{Lg}_{\mathrm{pu}}\,{\mathrm{Vbase}}^2}$
      | Automatically generated on 2025-10-09 21:36:40 .
  Input_v_d_GFL_17_26746 : Inport
  State_theta_pll_GFL_17_54061 : Inport  Port=2
  Input_v_q_GFL_17_9adff : Inport  Port=3
  State_theta_pll_GFL_17_ae1e4 : Inport  Port=4
  State_Iqv_GFL_17_7539a : Inport  Port=5
  State_i_gd_GFL_17_be3a3 : Inport  Port=6
  Input_v_d_GFL_17_c62dd : Inport  Port=7
  State_theta_pll_GFL_17_ade9f : Inport  Port=8
  Input_v_q_GFL_17_19e6b : Inport  Port=9
  State_theta_pll_GFL_17_5e05a : Inport  Port=10
  State_i_gq_GFL_17_952ec : Inport  Port=11
  Input_v_d_GFL_17_a9001 : Inport  Port=12
  State_theta_pll_GFL_17_c1a20 : Inport  Port=13
  Input_v_q_GFL_17_9c3f0 : Inport  Port=14
  State_theta_pll_GFL_17_d56bc : Inport  Port=15
  State_Phi_gc_GFL_17_446f2 : Inport  Port=16
  State_i_gq_GFL_17_272c2 : Inport  Port=17
  State_Phi_gd_GFL_17_5b911 : Inport  Port=18
  State_i_gq_GFL_17_921b2 : Inport  Port=19
  Add_30689 : Sum
  Add_47933 : Sum
  Add_7d88b : Sum
  Add_91d2a : Sum
  Add_ca3c8 : Sum
  Add_eb2f8 : Sum
  Constant_-1_df6a4 : Constant  Value=-1
  Constant_1.73205080756888_d9e20 : Constant  Value=1.73205080756888
  Constant_1.73205080756888_e7ae1 : Constant  Value=1.73205080756888
  Constant_2.0_7f0d8 : Constant  Value=2.0
  Constant_2.0_83778 : Constant  Value=2.0
  Constant_2.0_d4961 : Constant  Value=2.0
  Constant_Bva_41810 : Constant  Value=Bva
  Constant_Lg_pu_ff643 : Constant  Value=Lg_pu
  Constant_P_iq_1b39d : Constant  Value=P_iq
  Constant_P_oq_bf2cb : Constant  Value=P_oq
  Constant_Qe_ref_e2175 : Constant  Value=Qe_ref
  Constant_Rg_pu_30290 : Constant  Value=Rg_pu
  Constant_Sbase_a27b3 : Constant  Value=Sbase
  Constant_Sbase_a6581 : Constant  Value=Sbase
  Constant_Sbase_cef8a : Constant  Value=Sbase
  Constant_Vbase_2f635 : Constant  Value=Vbase
  Constant_Vbase_3abca : Constant  Value=Vbase
  Constant_Vbase_40423 : Constant  Value=Vbase
  Constant_Vbase_61625 : Constant  Value=Vbase
  Constant_Vbase_ed4d9 : Constant  Value=Vbase
  Constant_f0_4b851 : Constant  Value=f0
  Constant_pi_34f68 : Constant  Value=pi
  Divide_b6e15 : Product  Inputs=*/
  Divide_e9646 : Product  Inputs=*/
  MathFunc_cos_57582 : Trigonometry  Operator=cos
  MathFunc_cos_7ec7a : Trigonometry  Operator=cos
  MathFunc_cos_90985 : Trigonometry  Operator=cos
  MathFunc_sin_03ff8 : Trigonometry
  MathFunc_sin_1f042 : Trigonometry
  MathFunc_sin_715d0 : Trigonometry
  Power_678b0 : Math  Operator=pow
  Power_78a82 : Math  Operator=pow
  Product_0ddf2 : Product
  Product_149dd : Product
  Product_26735 : Product
  Product_27a96 : Product
  Product_2c204 : Product
  Product_359e4 : Product
  Product_406cf : Product
  Product_4095d : Product
  Product_476f9 : Product
  Product_49549 : Product
  Product_4a483 : Product
  Product_6d516 : Product
  Product_703bf : Product
  Product_74f61 : Product
  Product_81040 : Product
  Product_88e46 : Product
  Product_9150c : Product
  Product_99f51 : Product
  Product_adb80 : Product
  Product_b587c : Product
  Product_c3842 : Product
  Product_c8315 : Product
  Product_fe1cd : Product
  Product_ff042 : Product
  Product_fffc2 : Product
  Subtract_1fcb2 : Sum  Inputs=+-
  Subtract_34a5b : Sum  Inputs=+-
  Subtract_471d7 : Sum  Inputs=+-
  Subtract_5cfac : Sum  Inputs=+-
  Subtract_8a874 : Sum  Inputs=+-
  Blockout_d_i_gq_GFL_17_a2246 : Outport
  wires:
  State_theta_pll_GFL_17_ade9f/1 -> MathFunc_sin_715d0/1
  Input_v_q_GFL_17_9adff/1 -> Product_b587c/1
  State_theta_pll_GFL_17_5e05a/1 -> MathFunc_cos_7ec7a/1
  MathFunc_cos_7ec7a/1 -> Product_6d516/2
  Constant_Vbase_ed4d9/1 -> Product_81040/2
  State_i_gq_GFL_17_952ec/1 -> Product_0ddf2/2
  Product_81040/1 -> Product_27a96/1
  Constant_1.73205080756888_e7ae1/1 -> Product_81040/1
  Add_7d88b/1 -> Product_4095d/2
  Product_2c204/1 -> Add_ca3c8/1
  Input_v_d_GFL_17_c62dd/1 -> Product_2c204/1
  MathFunc_sin_715d0/1 -> Product_2c204/2
  Constant_Sbase_cef8a/1 -> Product_406cf/2
  Product_4095d/1 -> Add_eb2f8/1
  Product_6d516/1 -> Add_ca3c8/2
  Input_v_q_GFL_17_19e6b/1 -> Product_6d516/1
  Constant_Qe_ref_e2175/1 -> Product_703bf/2
  MathFunc_cos_57582/1 -> Product_74f61/2
  State_theta_pll_GFL_17_c1a20/1 -> MathFunc_cos_57582/1
  MathFunc_sin_03ff8/1 -> Product_c3842/2
  State_theta_pll_GFL_17_d56bc/1 -> MathFunc_sin_03ff8/1
  MathFunc_sin_1f042/1 -> Product_ff042/2
  State_theta_pll_GFL_17_54061/1 -> MathFunc_sin_1f042/1
  MathFunc_cos_90985/1 -> Product_b587c/2
  State_theta_pll_GFL_17_ae1e4/1 -> MathFunc_cos_90985/1
  Product_703bf/1 -> Product_406cf/1
  Constant_-1_df6a4/1 -> Product_703bf/1
  Product_ff042/1 -> Add_7d88b/1
  Product_149dd/1 -> Product_0ddf2/1
  Input_v_d_GFL_17_26746/1 -> Product_ff042/1
  Constant_1.73205080756888_d9e20/1 -> Product_149dd/1
  State_i_gd_GFL_17_be3a3/1 -> Product_27a96/2
  Constant_Bva_41810/1 -> Product_4a483/1
  Constant_Vbase_61625/1 -> Product_149dd/2
  Product_74f61/1 -> Subtract_8a874/1
  Input_v_d_GFL_17_a9001/1 -> Product_74f61/1
  Input_v_q_GFL_17_9c3f0/1 -> Product_c3842/1
  Product_27a96/1 -> Product_88e46/1
  Add_ca3c8/1 -> Product_88e46/2
  Product_c3842/1 -> Subtract_8a874/2
  Constant_Vbase_40423/1 -> Product_4a483/2
  Product_b587c/1 -> Add_7d88b/2
  Product_406cf/1 -> Subtract_5cfac/1
  Add_91d2a/1 -> Subtract_34a5b/1
  Product_88e46/1 -> Subtract_5cfac/2
  Product_0ddf2/1 -> Product_fffc2/1
  Subtract_8a874/1 -> Product_fffc2/2
  Product_4a483/1 -> Product_4095d/1
  Subtract_5cfac/1 -> Subtract_471d7/1
  State_Iqv_GFL_17_7539a/1 -> Add_eb2f8/2
  Product_fffc2/1 -> Subtract_471d7/2
  Constant_P_oq_bf2cb/1 -> Product_359e4/1
  Add_47933/1 -> Add_91d2a/1
  Subtract_471d7/1 -> Product_359e4/2
  Add_eb2f8/1 -> Add_47933/1
  Product_359e4/1 -> Add_47933/2
  State_Phi_gc_GFL_17_446f2/1 -> Add_91d2a/2
  Constant_2.0_83778/1 -> Power_678b0/2
  Constant_Vbase_3abca/1 -> Power_678b0/1
  State_i_gq_GFL_17_272c2/1 -> Subtract_34a5b/2
  Constant_Rg_pu_30290/1 -> Product_9150c/1
  Power_678b0/1 -> Product_9150c/2
  Constant_2.0_d4961/1 -> Product_476f9/1
  Product_adb80/1 -> Add_30689/1
  Constant_pi_34f68/1 -> Product_476f9/2
  Constant_P_iq_1b39d/1 -> Product_adb80/1
  Subtract_34a5b/1 -> Product_adb80/2
  Product_9150c/1 -> Product_99f51/1
  State_i_gq_GFL_17_921b2/1 -> Product_99f51/2
  Product_476f9/1 -> Product_fe1cd/1
  Constant_Sbase_a6581/1 -> Product_fe1cd/2
  State_Phi_gd_GFL_17_5b911/1 -> Add_30689/2
  Product_99f51/1 -> Divide_e9646/1
  Constant_Sbase_a27b3/1 -> Divide_e9646/2
  Product_fe1cd/1 -> Product_c8315/1
  Constant_f0_4b851/1 -> Product_c8315/2
  Add_30689/1 -> Subtract_1fcb2/1
  Divide_e9646/1 -> Subtract_1fcb2/2
  Subtract_1fcb2/1 -> Product_26735/2
  Constant_Vbase_2f635/1 -> Power_78a82/1
  Constant_2.0_7f0d8/1 -> Power_78a82/2
  Product_c8315/1 -> Product_26735/1
  Constant_Lg_pu_ff643/1 -> Product_49549/1
  Power_78a82/1 -> Product_49549/2
  Product_26735/1 -> Divide_b6e15/1
  Product_49549/1 -> Divide_b6e15/2
  Divide_b6e15/1 -> Blockout_d_i_gq_GFL_17_a2246/1

== system IEEE14_case/GFL_17/d_theta_pll_GFL_17_block ==
  note: d_theta_pll_GFL_17 in case14gfl
      | $\mathrm{Phipll}_{\mathrm{GFL},17}-P_{\mathrm{pll}}\,\left(\mathrm{vq}_{\mathrm{ref}}+v_{q,\mathrm{GFL},17}\,\cos\left(\theta _{\mathrm{pll},\mathrm{GFL},17}\right)+v_{d,\mathrm{GFL},17}\,\sin\left(\theta _{\mathrm{pll},\mathrm{GFL},17}\right)\right)$
      | Automatically generated on 2025-10-09 21:36:56 .
  Input_v_d_GFL_17_db4bf : Inport
  State_theta_pll_GFL_17_4c41d : Inport  Port=2
  Input_v_q_GFL_17_afffd : Inport  Port=3
  State_theta_pll_GFL_17_280fb : Inport  Port=4
  State_Phipll_GFL_17_89cae : Inport  Port=5
  Add_5a126 : Sum
  Constant_-1_720d0 : Constant  Value=-1
  Constant_P_pll_1564a : Constant  Value=P_pll
  Constant_vq_ref_73172 : Constant  Value=vq_ref
  MathFunc_cos_f3e74 : Trigonometry  Operator=cos
  MathFunc_sin_6d272 : Trigonometry
  Product_2d973 : Product
  Product_70c13 : Product
  Product_995fc : Product
  Product_ab8f6 : Product
  Subtract_aa56a : Sum  Inputs=+-
  Subtract_ebef4 : Sum  Inputs=+-
  Blockout_d_theta_pll_GFL_17_04ce6 : Outport
  wires:
  Constant_P_pll_1564a/1 -> Product_995fc/1
  MathFunc_cos_f3e74/1 -> Product_2d973/2
  Constant_-1_720d0/1 -> Product_ab8f6/1
  Product_ab8f6/1 -> Product_70c13/1
  Constant_vq_ref_73172/1 -> Subtract_aa56a/2
  Input_v_d_GFL_17_db4bf/1 -> Product_ab8f6/2
  State_theta_pll_GFL_17_4c41d/1 -> MathFunc_sin_6d272/1
  Product_70c13/1 -> Subtract_ebef4/1
  State_theta_pll_GFL_17_280fb/1 -> MathFunc_cos_f3e74/1
  MathFunc_sin_6d272/1 -> Product_70c13/2
  Input_v_q_GFL_17_afffd/1 -> Product_2d973/1
  Product_2d973/1 -> Subtract_ebef4/2
  Add_5a126/1 -> Blockout_d_theta_pll_GFL_17_04ce6/1
  Subtract_ebef4/1 -> Subtract_aa56a/1
  Product_995fc/1 -> Add_5a126/1
  Subtract_aa56a/1 -> Product_995fc/2
  State_Phipll_GFL_17_89cae/1 -> Add_5a126/2

== system IEEE14_case/GFL_17/e_dc_GFL_17_block ==
  note: e_dc_GFL_17 in case14gfl
      | $\frac{V_{\mathrm{dc},\mathrm{GFL},17}}{\mathrm{Vdcbase}}$
      | Automatically generated on 2025-10-09 21:37:14 .
  State_V_dc_GFL_17_df3ee : Inport
  Constant_Vdcbase_faab5 : Constant  Value=Vdcbase
  Divide_3931a : Product  Inputs=*/
  Blockout_e_dc_GFL_17_f966e : Outport
  wires:
  State_V_dc_GFL_17_df3ee/1 -> Divide_3931a/1
  Constant_Vdcbase_faab5/1 -> Divide_3931a/2
  Divide_3931a/1 -> Blockout_e_dc_GFL_17_f966e/1

== system IEEE14_case/GFL_17/i_d_GFL_17_block ==
  note: i_d_GFL_17 in case14gfl
      | $0.00658179306876173\,i_{\mathrm{gd},\mathrm{GFL},17}\,\cos\left(\theta _{\mathrm{pll},\mathrm{GFL},17}\right)+0.00658179306876173\,i_{\mathrm{gq},\mathrm{GFL},17}\,\sin\left(\theta _{\mathrm{pll},\mathrm{GFL},17}\right)$
      | Automatically generated on 2025-10-09 21:37:12 .
  State_i_gd_GFL_17_ef23a : Inport
  State_theta_pll_GFL_17_d2c5b : Inport  Port=2
  State_i_gq_GFL_17_23567 : Inport  Port=3
  State_theta_pll_GFL_17_5024c : Inport  Port=4
  Add_df983 : Sum
  Constant_0.00658179306876173_68133 : Constant  Value=0.00658179306876173
  Constant_0.00658179306876173_b16c1 : Constant  Value=0.00658179306876173
  MathFunc_cos_bdea1 : Trigonometry  Operator=cos
  MathFunc_sin_2c691 : Trigonometry
  Product_610b8 : Product
  Product_82ccf : Product
  Product_bf782 : Product
  Product_f147a : Product
  Blockout_i_d_GFL_17_3e529 : Outport
  wires:
  Constant_0.00658179306876173_b16c1/1 -> Product_610b8/1
  Product_610b8/1 -> Product_82ccf/1
  MathFunc_sin_2c691/1 -> Product_bf782/2
  State_theta_pll_GFL_17_5024c/1 -> MathFunc_sin_2c691/1
  State_theta_pll_GFL_17_d2c5b/1 -> MathFunc_cos_bdea1/1
  Add_df983/1 -> Blockout_i_d_GFL_17_3e529/1
  State_i_gd_GFL_17_ef23a/1 -> Product_610b8/2
  Constant_0.00658179306876173_68133/1 -> Product_f147a/1
  State_i_gq_GFL_17_23567/1 -> Product_f147a/2
  MathFunc_cos_bdea1/1 -> Product_82ccf/2
  Product_f147a/1 -> Product_bf782/1
  Product_82ccf/1 -> Add_df983/1
  Product_bf782/1 -> Add_df983/2

== system IEEE14_case/GFL_17/i_q_GFL_17_block ==
  note: i_q_GFL_17 in case14gfl
      | $0.00658179306876173\,i_{\mathrm{gq},\mathrm{GFL},17}\,\cos\left(\theta _{\mathrm{pll},\mathrm{GFL},17}\right)-0.00658179306876173\,i_{\mathrm{gd},\mathrm{GFL},17}\,\sin\left(\theta _{\mathrm{pll},\mathrm{GFL},17}\right)$
      | Automatically generated on 2025-10-09 21:37:13 .
  State_i_gd_GFL_17_b074d : Inport
  State_theta_pll_GFL_17_da001 : Inport  Port=2
  State_i_gq_GFL_17_4b654 : Inport  Port=3
  State_theta_pll_GFL_17_5726e : Inport  Port=4
  Add_dda6a : Sum
  Constant_-0.00658179306876173_8d86e : Constant  Value=-0.00658179306876173
  Constant_0.00658179306876173_3cc02 : Constant  Value=0.00658179306876173
  MathFunc_cos_2b9aa : Trigonometry  Operator=cos
  MathFunc_sin_414d0 : Trigonometry
  Product_30e67 : Product
  Product_68b9b : Product
  Product_8c178 : Product
  Product_b1e97 : Product
  Blockout_i_q_GFL_17_34d19 : Outport
  wires:
  Constant_-0.00658179306876173_8d86e/1 -> Product_68b9b/1
  Constant_0.00658179306876173_3cc02/1 -> Product_8c178/1
  State_i_gd_GFL_17_b074d/1 -> Product_68b9b/2
  State_theta_pll_GFL_17_da001/1 -> MathFunc_sin_414d0/1
  MathFunc_sin_414d0/1 -> Product_30e67/2
  MathFunc_cos_2b9aa/1 -> Product_b1e97/2
  State_theta_pll_GFL_17_5726e/1 -> MathFunc_cos_2b9aa/1
  State_i_gq_GFL_17_4b654/1 -> Product_8c178/2
  Product_68b9b/1 -> Product_30e67/1
  Product_8c178/1 -> Product_b1e97/1
  Product_30e67/1 -> Add_dda6a/1
  Product_b1e97/1 -> Add_dda6a/2
  Add_dda6a/1 -> Blockout_i_q_GFL_17_34d19/1

== system IEEE14_case/GFL_18/d_Idv_GFL_18_block ==
  note: d_Idv_GFL_18 in case14gfl
      | $-\frac{\mathrm{Idv}_{\mathrm{GFL},18}+\mathrm{Kdo}\,\left(\mathrm{Vbase}\,\left(v_{q,\mathrm{GFL},18}\,\cos\left(\theta _{\mathrm{pll},\mathrm{GFL},18}\right)+v_{d,\mathrm{GFL},18}\,\sin\left(\theta _{\mathrm{pll},\mathrm{GFL},18}\right)\right)+\frac{\Psi _{d,\mathrm{GFL},18}+\mathrm{Kdi}\,\mathrm{Vbase}\,\left(v_{q,\mathrm{GFL},18}\,\cos\left(\theta _{\mathrm{pll},\mathrm{GFL},18}\right)+v_{d,\mathrm{GFL},18}\,\sin\left(\theta _{\mathrm{pll},\mathrm{GFL},18}\right)\right)}{\mathrm{Tdi}}\right)}{\mathrm{Tdo}}$
      | Automatically generated on 2025-10-09 21:38:01 .
  State_Idv_GFL_18_af2bb : Inport
  Input_v_d_GFL_18_10cbd : Inport  Port=2
  State_theta_pll_GFL_18_4128c : Inport  Port=3
  Input_v_q_GFL_18_fc279 : Inport  Port=4
  State_theta_pll_GFL_18_96f6a : Inport  Port=5
  Input_v_d_GFL_18_0ae0e : Inport  Port=6
  State_theta_pll_GFL_18_4866f : Inport  Port=7
  Input_v_q_GFL_18_9cb7b : Inport  Port=8
  State_theta_pll_GFL_18_af8c5 : Inport  Port=9
  State_Psi_d_GFL_18_c430f : Inport  Port=10
  Add_0a0f3 : Sum
  Add_6a636 : Sum
  Add_9bb4b : Sum
  Add_fb9a2 : Sum
  Constant_-1_07302 : Constant  Value=-1
  Constant_-1_d1c32 : Constant  Value=-1
  Constant_-1_f225f : Constant  Value=-1
  Constant_Kdi_9348d : Constant  Value=Kdi
  Constant_Kdo_372d1 : Constant  Value=Kdo
  Constant_Tdi_fec6a : Constant  Value=Tdi
  Constant_Tdo_3de8e : Constant  Value=Tdo
  Constant_Vbase_3fc23 : Constant  Value=Vbase
  Constant_Vbase_5d08c : Constant  Value=Vbase
  Divide_b6b0d : Product  Inputs=*/
  Divide_ccc37 : Product  Inputs=*/
  MathFunc_cos_1f766 : Trigonometry  Operator=cos
  MathFunc_cos_6715f : Trigonometry  Operator=cos
  MathFunc_sin_ace9a : Trigonometry
  MathFunc_sin_c51e6 : Trigonometry
  Product_0353f : Product
  Product_15237 : Product
  Product_5d7a6 : Product
  Product_6b26f : Product
  Product_6df7a : Product
  Product_94ad9 : Product
  Product_9d3f5 : Product
  Product_af73a : Product
  Product_bb2c7 : Product
  Product_ccd2f : Product
  Product_e370f : Product
  Subtract_4a344 : Sum  Inputs=+-
  Blockout_d_Idv_GFL_18_15e6a : Outport
  wires:
  State_theta_pll_GFL_18_4866f/1 -> MathFunc_sin_ace9a/1
  MathFunc_sin_ace9a/1 -> Product_bb2c7/2
  Constant_Tdo_3de8e/1 -> Divide_b6b0d/2
  Input_v_d_GFL_18_0ae0e/1 -> Product_bb2c7/1
  State_theta_pll_GFL_18_af8c5/1 -> MathFunc_cos_6715f/1
  Product_af73a/1 -> Product_ccd2f/1
  Constant_-1_d1c32/1 -> Product_af73a/1
  Constant_Vbase_3fc23/1 -> Product_ccd2f/2
  Constant_Kdi_9348d/1 -> Product_af73a/2
  MathFunc_cos_6715f/1 -> Product_9d3f5/2
  Input_v_q_GFL_18_9cb7b/1 -> Product_9d3f5/1
  State_theta_pll_GFL_18_4128c/1 -> MathFunc_sin_c51e6/1
  Product_5d7a6/1 -> Add_0a0f3/1
  State_theta_pll_GFL_18_96f6a/1 -> MathFunc_cos_1f766/1
  Add_9bb4b/1 -> Product_6df7a/2
  Product_bb2c7/1 -> Add_9bb4b/1
  Product_9d3f5/1 -> Add_9bb4b/2
  Product_6b26f/1 -> Add_fb9a2/2
  Constant_Kdo_372d1/1 -> Product_6b26f/1
  Input_v_d_GFL_18_10cbd/1 -> Product_0353f/1
  MathFunc_sin_c51e6/1 -> Product_0353f/2
  Product_15237/1 -> Add_6a636/2
  Input_v_q_GFL_18_fc279/1 -> Product_15237/1
  Add_0a0f3/1 -> Product_6b26f/2
  MathFunc_cos_1f766/1 -> Product_15237/2
  Product_6df7a/1 -> Subtract_4a344/1
  Product_ccd2f/1 -> Product_6df7a/1
  Product_94ad9/1 -> Product_5d7a6/1
  Constant_-1_f225f/1 -> Product_94ad9/1
  Constant_Vbase_5d08c/1 -> Product_94ad9/2
  Add_6a636/1 -> Product_5d7a6/2
  Product_0353f/1 -> Add_6a636/1
  State_Psi_d_GFL_18_c430f/1 -> Subtract_4a344/2
  Divide_ccc37/1 -> Add_0a0f3/2
  Subtract_4a344/1 -> Divide_ccc37/1
  Constant_Tdi_fec6a/1 -> Divide_ccc37/2
  Constant_-1_07302/1 -> Product_e370f/1
  State_Idv_GFL_18_af2bb/1 -> Product_e370f/2
  Product_e370f/1 -> Add_fb9a2/1
  Add_fb9a2/1 -> Divide_b6b0d/1
  Divide_b6b0d/1 -> Blockout_d_Idv_GFL_18_15e6a/1

== system IEEE14_case/GFL_18/d_Iqv_GFL_18_block ==
  note: d_Iqv_GFL_18 in case14gfl
      | $-\frac{\mathrm{Iqv}_{\mathrm{GFL},18}-\mathrm{Kqo}\,\left(\mathrm{Vbase}\,\left(v_{d,\mathrm{GFL},18}\,\cos\left(\theta _{\mathrm{pll},\mathrm{GFL},18}\right)-v_{q,\mathrm{GFL},18}\,\sin\left(\theta _{\mathrm{pll},\mathrm{GFL},18}\right)\right)-\frac{\Psi _{q,\mathrm{GFL},18}-\mathrm{Kqi}\,\mathrm{Vbase}\,\left(v_{d,\mathrm{GFL},18}\,\cos\left(\theta _{\mathrm{pll},\mathrm{GFL},18}\right)-v_{q,\mathrm{GFL},18}\,\sin\left(\theta _{\mathrm{pll},\mathrm{GFL},18}\right)\right)}{\mathrm{Tqi}}\right)}{\mathrm{Tqo}}$
      | Automatically generated on 2025-10-09 21:38:03 .
  State_Iqv_GFL_18_dba96 : Inport
  Input_v_d_GFL_18_b6341 : Inport  Port=2
  State_theta_pll_GFL_18_8f911 : Inport  Port=3
  Input_v_q_GFL_18_86533 : Inport  Port=4
  State_theta_pll_GFL_18_b687b : Inport  Port=5
  Input_v_d_GFL_18_59aa3 : Inport  Port=6
  State_theta_pll_GFL_18_7a1d2 : Inport  Port=7
  Input_v_q_GFL_18_04b2f : Inport  Port=8
  State_theta_pll_GFL_18_15ee8 : Inport  Port=9
  State_Psi_q_GFL_18_f1020 : Inport  Port=10
  Add_1972a : Sum
  Add_78d7c : Sum
  Constant_-1_6f3c1 : Constant  Value=-1
  Constant_Kqi_e2fe0 : Constant  Value=Kqi
  Constant_Kqo_de095 : Constant  Value=Kqo
  Constant_Tqi_8925b : Constant  Value=Tqi
  Constant_Tqo_427c0 : Constant  Value=Tqo
  Constant_Vbase_b2bf8 : Constant  Value=Vbase
  Constant_Vbase_be836 : Constant  Value=Vbase
  Divide_8c24d : Product  Inputs=*/
  Divide_9a55d : Product  Inputs=*/
  MathFunc_cos_1f264 : Trigonometry  Operator=cos
  MathFunc_cos_2e4c7 : Trigonometry  Operator=cos
  MathFunc_sin_e4898 : Trigonometry
  MathFunc_sin_e5c77 : Trigonometry
  Product_111ae : Product
  Product_16019 : Product
  Product_2c96f : Product
  Product_65651 : Product
  Product_7b2e8 : Product
  Product_a8345 : Product
  Product_bafca : Product
  Product_db37c : Product
  Product_db7db : Product
  Subtract_4c73f : Sum  Inputs=+-
  Subtract_98895 : Sum  Inputs=+-
  Subtract_c58c7 : Sum  Inputs=+-
  Blockout_d_Iqv_GFL_18_c4d55 : Outport
  wires:
  MathFunc_cos_1f264/1 -> Product_db7db/2
  State_theta_pll_GFL_18_8f911/1 -> MathFunc_cos_1f264/1
  State_theta_pll_GFL_18_7a1d2/1 -> MathFunc_cos_2e4c7/1
  MathFunc_cos_2e4c7/1 -> Product_111ae/2
  MathFunc_sin_e5c77/1 -> Product_65651/2
  State_theta_pll_GFL_18_b687b/1 -> MathFunc_sin_e5c77/1
  State_theta_pll_GFL_18_15ee8/1 -> MathFunc_sin_e4898/1
  MathFunc_sin_e4898/1 -> Product_db37c/2
  Constant_Tqi_8925b/1 -> Divide_9a55d/2
  Product_111ae/1 -> Subtract_98895/1
  Input_v_d_GFL_18_59aa3/1 -> Product_111ae/1
  Product_db37c/1 -> Subtract_98895/2
  Input_v_q_GFL_18_04b2f/1 -> Product_db37c/1
  Product_a8345/1 -> Add_1972a/1
  Product_16019/1 -> Product_7b2e8/1
  Constant_Kqi_e2fe0/1 -> Product_16019/1
  Constant_Vbase_b2bf8/1 -> Product_16019/2
  Product_db7db/1 -> Subtract_c58c7/1
  Input_v_d_GFL_18_b6341/1 -> Product_db7db/1
  Product_65651/1 -> Subtract_c58c7/2
  Input_v_q_GFL_18_86533/1 -> Product_65651/1
  Product_2c96f/1 -> Add_78d7c/2
  Product_bafca/1 -> Add_78d7c/1
  Subtract_98895/1 -> Product_7b2e8/2
  Subtract_4c73f/1 -> Divide_9a55d/1
  Product_7b2e8/1 -> Subtract_4c73f/1
  State_Psi_q_GFL_18_f1020/1 -> Subtract_4c73f/2
  Constant_Vbase_be836/1 -> Product_a8345/1
  Subtract_c58c7/1 -> Product_a8345/2
  Divide_9a55d/1 -> Add_1972a/2
  Constant_-1_6f3c1/1 -> Product_bafca/1
  State_Iqv_GFL_18_dba96/1 -> Product_bafca/2
  Constant_Kqo_de095/1 -> Product_2c96f/1
  Add_1972a/1 -> Product_2c96f/2
  Add_78d7c/1 -> Divide_8c24d/1
  Constant_Tqo_427c0/1 -> Divide_8c24d/2
  Divide_8c24d/1 -> Blockout_d_Iqv_GFL_18_c4d55/1

== system IEEE14_case/GFL_18/d_Phi_ga_GFL_18_block ==
  note: d_Phi_ga_GFL_18 in case14gfl
      | $I_{\mathrm{od}}\,\left(V_{\mathrm{dc},\mathrm{GFL},18}-\mathrm{Vdcbase}\,\mathrm{Vdc}_{\mathrm{ref}}\right)$
      | Automatically generated on 2025-10-09 21:37:48 .
  State_V_dc_GFL_18_2da35 : Inport
  Constant_I_od_06755 : Constant  Value=I_od
  Constant_Vdc_ref_9a016 : Constant  Value=Vdc_ref
  Constant_Vdcbase_0561a : Constant  Value=Vdcbase
  Product_0fd9f : Product
  Product_d8266 : Product
  Subtract_ddee2 : Sum  Inputs=+-
  Blockout_d_Phi_ga_GFL_18_9b191 : Outport
  wires:
  Product_0fd9f/1 -> Subtract_ddee2/2
  Constant_Vdc_ref_9a016/1 -> Product_0fd9f/1
  Constant_Vdcbase_0561a/1 -> Product_0fd9f/2
  State_V_dc_GFL_18_2da35/1 -> Subtract_ddee2/1
  Constant_I_od_06755/1 -> Product_d8266/1
  Subtract_ddee2/1 -> Product_d8266/2
  Product_d8266/1 -> Blockout_d_Phi_ga_GFL_18_9b191/1
